simulink model "TexomaHomeEducatorsRobotProgram"  (R2019b)
settings: Solver=FixedStepAuto  StartTime=0.0  StopTime=10.0  RelTol=1e-3
libraries: vexarmcortexlib x15, vexcommonlib x2
settings Model: ExtModeTrigDuration=25  Creator=jakew  LastModifiedBy=brigh
settings OptimizationCC: EnhancedBackFolding=on  PassReuseOutputArgsAs=Individual arguments  ZeroExternalMemoryAtStartup=off  ZeroInternalMemoryAtStartup=off  MaxStackSize=64  OptimizeBlockOrder=speed  DifferentSizesBufferReuse=on  OptimizationCustomize=off  EfficientTunableParamExpr=on
settings DebuggingCC: ParameterTunabilityLossMsg=error
settings HardwareCC: ProdBitPerPointer=32  ProdBitPerSizeT=32  ProdBitPerPtrDiffT=32  ProdLargestAtomicInteger=Long  ProdLargestAtomicFloat=Double  ProdWordSize=32  ProdHWDeviceType=ARM Compatible->ARM Cortex
settings SFSimCC: MATLABDynamicMemAlloc=off
settings RTWCC: SystemTargetFile=ert.tlc  HardwareBoard=ARM Cortex-based VEX Microcontroller  TLCOptions="-aInlineSetEventsForThisBaseRateFcn=TLC_FALSE -aSuppressMultiTaskScheduler=TLC_FALSE  -aRateBasedStepFcn=0"  TemplateMakefile=ert_default_tmf  GenerateReport=on  Toolchain=GNU Tools for VEX ARM Cortex  IncludeHyperlinkInReport=on  LaunchReport=on  GenerateTraceInfo=on  GenerateTraceReport=on  GenerateTraceReportSl=on  GenerateTraceReportSf=on  GenerateTraceReportEml=on
settings CodeAppCC: ForceParamTrailComments=on  IgnoreCustomStorageClasses=off  OperatorAnnotations=on  SimulinkDataObjDesc=on  SFDataObjDesc=on  InsertBlockDesc=on

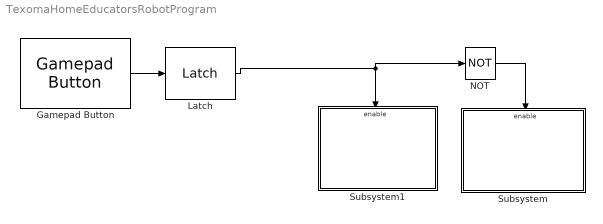
== system TexomaHomeEducatorsRobotProgram ==
  Gamepad Button : vexarmcortexlib/Gamepad/Gamepad Button  joystick=1  chan=7  button56=Up  button78=Up  SimulationIn=off  SampleTime=0.02
      settings: SourceProductName=Simulink Coder Support Package for ARM Cortex-based VEX Microcontroller  SourceProductBaseCode=EC_VEX_MICRO
  Latch : vexcommonlib/Latch  output0=off  BlockPlatform=vexarmcortex
      settings: SourceProductName=Simulink Coder Support Package for ARM Cortex-based VEX Microcontroller  SourceProductBaseCode=EC_VEX_MICRO
  NOT : Logic  Operator=NOT  IconShape=distinctive  AllPortsSameDT=off  OutDataTypeStr=boolean
  Subsystem : Subsystem
  Subsystem1 : Subsystem
  wires:
  Gamepad Button/1 -> Latch/1
  Latch/1 -> Subsystem1/Enable, NOT/1
  NOT/1 -> Subsystem/Enable

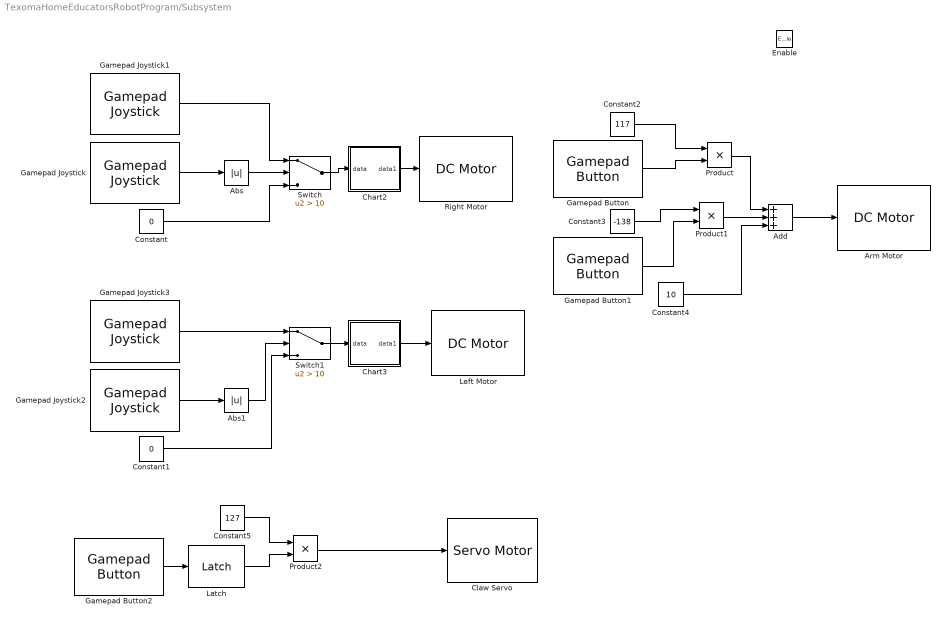
== system TexomaHomeEducatorsRobotProgram/Subsystem ==
  Enable : EnablePort
  Abs : Abs
  Abs1 : Abs
  Add : Sum  Inputs=+++
  "Arm Motor " : vexarmcortexlib/Actuators/DC Motor  motor=8  scaleFactor=1/13.5  SimulationOut=off
      settings: SourceProductName=Simulink Coder Support Package for ARM Cortex-based VEX Microcontroller  SourceProductBaseCode=EC_VEX_MICRO
  Chart2 : Stateflow chart  BlockKeywords=__PRM__SERIALIZED__DATA__:Stateflow Chart,Stateflow Diagram  TreatAsAtomicUnit=on
  Chart3 : Stateflow chart  BlockKeywords=__PRM__SERIALIZED__DATA__:Stateflow Chart,Stateflow Diagram  TreatAsAtomicUnit=on
  Claw Servo : vexarmcortexlib/Actuators/Servo Motor  motor=9  scaleFactor=60/127  SimulationOut=off
      settings: SourceProductName=Simulink Coder Support Package for ARM Cortex-based VEX Microcontroller  SourceProductBaseCode=EC_VEX_MICRO
  Constant : Constant  Value=0
  Constant1 : Constant  Value=0
  Constant2 : Constant  Value=117
  Constant3 : Constant  Value=-138
  Constant4 : Constant  Value=10
  Constant5 : Constant  Value=127
  Gamepad Button : vexarmcortexlib/Gamepad/Gamepad Button  joystick=1  chan=6  button56=Up  button78=Down  SimulationIn=off  SampleTime=0.02
      settings: SourceProductName=Simulink Coder Support Package for ARM Cortex-based VEX Microcontroller  SourceProductBaseCode=EC_VEX_MICRO
  Gamepad Button1 : vexarmcortexlib/Gamepad/Gamepad Button  joystick=1  chan=6  button56=Down  button78=Down  SimulationIn=off  SampleTime=0.02
      settings: SourceProductName=Simulink Coder Support Package for ARM Cortex-based VEX Microcontroller  SourceProductBaseCode=EC_VEX_MICRO
  Gamepad Button2 : vexarmcortexlib/Gamepad/Gamepad Button  joystick=1  chan=5  button56=Up  button78=Down  SimulationIn=off  SampleTime=0.02
      settings: SourceProductName=Simulink Coder Support Package for ARM Cortex-based VEX Microcontroller  SourceProductBaseCode=EC_VEX_MICRO
  Gamepad Joystick : vexarmcortexlib/Gamepad/Gamepad Joystick  joystick=1  chan=2  SimulationIn=off  SampleTime=0.02
      settings: SourceProductName=Simulink Coder Support Package for ARM Cortex-based VEX Microcontroller  SourceProductBaseCode=EC_VEX_MICRO
  Gamepad Joystick1 : vexarmcortexlib/Gamepad/Gamepad Joystick  joystick=1  chan=2  SimulationIn=off  SampleTime=0.02
      settings: SourceProductName=Simulink Coder Support Package for ARM Cortex-based VEX Microcontroller  SourceProductBaseCode=EC_VEX_MICRO
  Gamepad Joystick2 : vexarmcortexlib/Gamepad/Gamepad Joystick  joystick=1  chan=3  SimulationIn=off  SampleTime=0.02
      settings: SourceProductName=Simulink Coder Support Package for ARM Cortex-based VEX Microcontroller  SourceProductBaseCode=EC_VEX_MICRO
  Gamepad Joystick3 : vexarmcortexlib/Gamepad/Gamepad Joystick  joystick=1  chan=3  SimulationIn=off  SampleTime=0.02
      settings: SourceProductName=Simulink Coder Support Package for ARM Cortex-based VEX Microcontroller  SourceProductBaseCode=EC_VEX_MICRO
  Latch : vexcommonlib/Latch  output0=off  BlockPlatform=vexarmcortex
      settings: SourceProductName=Simulink Coder Support Package for ARM Cortex-based VEX Microcontroller  SourceProductBaseCode=EC_VEX_MICRO
  Left Motor : vexarmcortexlib/Actuators/DC Motor  motor=3  scaleFactor=1/13.5  SimulationOut=off
      settings: SourceProductName=Simulink Coder Support Package for ARM Cortex-based VEX Microcontroller  SourceProductBaseCode=EC_VEX_MICRO
  Product : Product
  Product1 : Product
  Product2 : Product
  Right Motor : vexarmcortexlib/Actuators/DC Motor  motor=2  scaleFactor=1/13.5  SimulationOut=off
      settings: SourceProductName=Simulink Coder Support Package for ARM Cortex-based VEX Microcontroller  SourceProductBaseCode=EC_VEX_MICRO
  Switch : Switch  Criteria=u2 > Threshold  Threshold=10
  Switch1 : Switch  Criteria=u2 > Threshold  Threshold=10
  wires:
  Gamepad Joystick2/1 -> Abs1/1
  Switch1/1 -> Chart3/1(data)
  Gamepad Joystick/1 -> Abs/1
  Constant3/1 -> Product1/1
  Add/1 -> "Arm Motor "/1
  Product2/1 -> Claw Servo/1
  Abs1/1 -> Switch1/2
  Gamepad Button/1 -> Product/2
  Product1/1 -> Add/2
  Constant4/1 -> Add/3
  Constant1/1 -> Switch1/3
  Gamepad Button1/1 -> Product1/2
  Constant/1 -> Switch/3
  Product/1 -> Add/1
  Constant5/1 -> Product2/1
  Switch/1 -> Chart2/1(data)
  Latch/1 -> Product2/2
  Gamepad Button2/1 -> Latch/1
  Gamepad Joystick1/1 -> Switch/1
  Constant2/1 -> Product/1
  Abs/1 -> Switch/2
  Gamepad Joystick3/1 -> Switch1/1
  Chart2/1(data1) -> Right Motor/1
  Chart3/1(data1) -> Left Motor/1

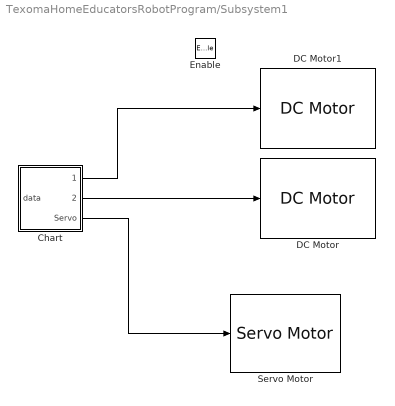
== system TexomaHomeEducatorsRobotProgram/Subsystem1 ==
  Enable : EnablePort
  Chart : Stateflow chart  BlockKeywords=__PRM__SERIALIZED__DATA__:Stateflow Chart,Stateflow Diagram  TreatAsAtomicUnit=on
  DC Motor : vexarmcortexlib/Actuators/DC Motor  motor=3  scaleFactor=1/13.5  SimulationOut=off
      settings: SourceProductName=Simulink Coder Support Package for ARM Cortex-based VEX Microcontroller  SourceProductBaseCode=EC_VEX_MICRO
  DC Motor1 : vexarmcortexlib/Actuators/DC Motor  motor=2  scaleFactor=1/13.5  SimulationOut=off
      settings: SourceProductName=Simulink Coder Support Package for ARM Cortex-based VEX Microcontroller  SourceProductBaseCode=EC_VEX_MICRO
  Servo Motor : vexarmcortexlib/Actuators/Servo Motor  motor=9  scaleFactor=60/127  SimulationOut=off
      settings: SourceProductName=Simulink Coder Support Package for ARM Cortex-based VEX Microcontroller  SourceProductBaseCode=EC_VEX_MICRO
  wires:
  Chart/3(Servo) -> Servo Motor/1
  Chart/1(Rspeed) -> DC Motor1/1
  Chart/2(Lspeed) -> DC Motor/1

== stateflow chart TexomaHomeEducatorsRobotProgram/Subsystem/Chart3 ==
  state Drive_Forward
    during: Lspeed=125;
  (default) -> Drive_Forward : {Lspeed=0;}
  data: data input; data1 output

== stateflow chart TexomaHomeEducatorsRobotProgram/Subsystem1/Chart ==
  state Drive_Forward
    during: Lspeed=125;
    during: Rspeed=100;
  state Stop1
    during:Lspeed=0;
    during:Rspeed=-0;
  state Release
    during:Lspeed=0;
    during:Rspeed=0;
    during:Servo=0;
  state Stop
    during:Lspeed=0;
    during:Rspeed=0;
    during:Servo=127;
  state Move_Back
    during:Lspeed=-125;
    during:Rspeed=-100;
  (default) -> Drive_Forward : {Lspeed=0; Rspeed=0; Servo=127;}
  Stop -> Drive_Forward : after(5,sec)
  Drive_Forward -> Stop1 : after(2.5,sec)
  Stop1 -> Release : after(.5,sec)
  Release -> Move_Back : after(.5,sec)
  Move_Back -> Stop : after(1,sec)
  data: Rspeed output; Lspeed output; Servo output; data input

== stateflow chart TexomaHomeEducatorsRobotProgram/Subsystem/Chart2 ==
  state Drive_Forward
    during: Rspeed=100;
  (default) -> Drive_Forward : {Rspeed=0;}
  data: data input; data1 output
